simulink model "Lift_Hierarchial_Model"  (R2020b)
settings: Solver=VariableStepAuto  StartTime=0.0  StopTime=10.0  RelTol=1e-3
settings Model: Creator=Manoj  LastModifiedBy=Windows 10

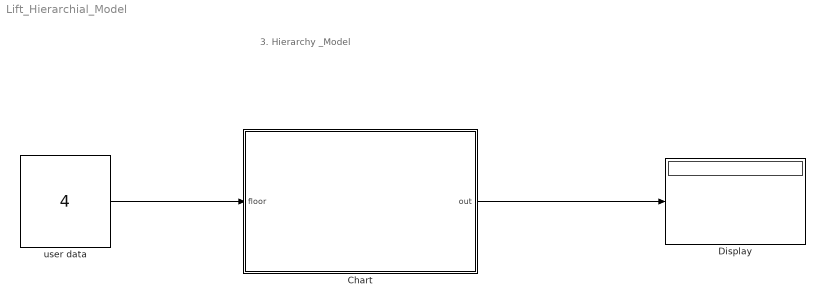
== system Lift_Hierarchial_Model ==
  note: 3. Hierarchy _Model
  Chart : Stateflow chart  TreatAsAtomicUnit=on
  Display : Display
  user data : Constant  Value=4
  wires:
  user data/1 -> Chart/1(floor)
  Chart/1(out) -> Display/1

== stateflow chart Lift_Hierarchial_Model/Chart ==
  state active
    state stop
      out=current;
    state down
      entry:
      current=current-1;
      out=current;
    state up
      entry:
      current=current+1;
      out=current;
    stop -> stop [order 1] : [floor==current]
    (default) -> stop
    stop -> up [order 2] : [current<floor]
    stop -> down [order 3] : [current>floor]
    up -> stop [order 1] : [current==floor]
    down -> stop : [current==floor]
    up -> up [order 2] : [current<floor]
  state wait
    entry:
    count=0;
    during:
    count=count+1;
  (default) -> active : {current=0;}
  (junction 19) -> stop [order 3]
  (junction 19) -> up [order 1] : [current<floor]
  (junction 19) -> down [order 2] : [current>floor]
  active -> wait : [current~=floor]
  wait -> (junction 19) : [count==2]
  data: out output; count local; current local =1; floor input
